simulink model "GTPR_OpenLoop"  (R2021a)
settings: Solver=ode4  StartTime=0.0  StopTime=t_end  FixedStep=t_step  RelTol=1e-3  AbsTol=1e-3
model workspace (MAT data in the model file):
  dt_planner = 0.001
  dt_solver = 0.0002
values from neighbouring files (symbols this model uses):
  aA = 0.5    [SimMechanics_GTPR_OpenLoop_CircularMotion_VS_ClosedLoop.m]
  aB = 0.5    [SimMechanics_GTPR_OpenLoop_CircularMotion_VS_ClosedLoop.m]
  aC = 0.5    [SimMechanics_GTPR_OpenLoop_CircularMotion_VS_ClosedLoop.m]
  dq_init = dq_des_c(:,1)    [SimMechanics_GTPR_OpenLoop_CircularMotion_VS_ClosedLoop.m]
  eA = 0.28    [SimMechanics_GTPR_OpenLoop_CircularMotion_VS_ClosedLoop.m]
  eB = 0.28    [SimMechanics_GTPR_OpenLoop_CircularMotion_VS_ClosedLoop.m]
  eC = 0.28    [SimMechanics_GTPR_OpenLoop_CircularMotion_VS_ClosedLoop.m]
  ILA = zeros(3)    [SimMechanics_GTPR_OpenLoop_CircularMotion_VS_ClosedLoop.m]
  IlA = zeros(3)    [SimMechanics_GTPR_OpenLoop_CircularMotion_VS_ClosedLoop.m]
  ILB = zeros(3)    [SimMechanics_GTPR_OpenLoop_CircularMotion_VS_ClosedLoop.m]
  IlB = zeros(3)    [SimMechanics_GTPR_OpenLoop_CircularMotion_VS_ClosedLoop.m]
  ILC = zeros(3)    [SimMechanics_GTPR_OpenLoop_CircularMotion_VS_ClosedLoop.m]
  q_init = q_des_c(:,1)    [SimMechanics_GTPR_OpenLoop_CircularMotion_VS_ClosedLoop.m]
  t_step = 0.001    [SimMechanics_GTPR_OpenLoop_CircularMotion_VS_ClosedLoop.m]
libraries: nesl_utility x22, sm_lib x3, GTPR_Library x1
CloseFcn:
  | clear sm_pick_and_place_robot_ik
  | clear sm_pick_and_place_robot_fk
Description:
  | Pick and Place Robot with Forward and Inverse Kinematics
settings Model: Creator=The MathWorks, Inc.  LastModifiedBy=szucs
settings SolverCC: NumberNewtonIterations=100  AlgebraicLoopSolver=TrustRegion
settings DataIOCC: ReturnWorkspaceOutputs=off
settings DebuggingCC: SFMachineParentedDataDiag=warning
settings SimscapeCC: SimscapeLogType=all  SimscapeLogSimulationStatistics=on  SimscapeLogName=simlog_sm_pick_and_place_robot  SimscapeLogDataHistory=10000
settings ExplorerConfigSet: InternalSimMechanicsExplorerSettings="<ExplorerConfiguration><canonicalview>default</canonicalview><AnimationSetting><BasePlaybackSpeed>1.0</BasePlaybackSpeed><PlaybackSpeedFactor>1.0</PlaybackSpeedFactor></AnimationSetting><TilePanel><TileInfo><Tiles Columns=\"2\" Count=\"3\" Rows=\"2\"><Column Weight=\"0.5\"/><Column Weight=\"0.5\"/><Row Weight=\"0.3038\"/><Row Weight=\"0.6962\"/><Tile Height=\"2\" Width=\"1\" X=\"0\" Y=\"0\"/><Tile Height=\"1\" Width=\"1\" X=\"1\" Y=\"0\"/><Tile Height=\"1\" Width=\"1\" X=\"1\" Y=\"1\"/></Tiles></TileInfo><SceneInfo><SceneViewer><BGColor><R>0.60000002384185791</R><G>0.60000002384185791</G><B>0.60000002384185791</B></BGColor><Camera><DoPerspective>off</DoPerspective><Position><X>0.674555883500480347</X><Y>-0.674555883500480902</Y><Z>0.921885249943208973</Z></Position><Center><X>0.0060149771328419227</X><Y>-0.00601497713284246394</Y><Z>0.253344343575570674</Z></Center><Up><X>-0.408248290463863073</X><Y>0.408248290463863073</Y><Z>0.816496580927726145</Z></Up><ViewLimDist>1</ViewLimDist><YLim>0.43506960332393646</YLim><XLim>0.392966093324845833</XLim></Camera></SceneViewer><SceneViewer><BGColor><R>0.60000002384185791</R><G>0.60000002384185791</G><B>0.60000002384185791</B></BGColor><Camera><DoPerspective>off</DoPerspective><Position><X>-0.000385309004919674389</X><Y>-1.33915517216324798</Y><Z>0.0518624305243804845</Z></Position><Center><X>-0.000385309004919674389</X><Y>0.0454699993133544367</Y><Z>0.0518624305243804845</Z></Center><Up><X>0</X><Y>-0</Y><Z>1</Z></Up><ViewLimDist>1</ViewLimDist><YLim>0.0894075615531887413</YLim><XLim>0.282074560393158813</XLim></Camera></SceneViewer><SceneViewer><BGColor><R>0.60000002384185791</R><G>0.60000002384185791</G><B>0.60000002384185791</B></BGColor><Camera><DoPerspective>on</DoPerspective><Position><X>-1.13755508710961844e-18</X><Y>-8.63362207815730793e-18</Y><Z>0.589999999999999969</Z></Position><Center><X>-1.13755508710961844e-18</X><Y>-8.63362207815730793e-18</Y><Z>-0.410000000000000031</Z></Center><Up><X>0</X><Y>1</Y><Z>0</Z></Up><ViewLimDist>1</ViewLimDist><YLim>0.466307658154998583</YLim><XLim>0.621743544206664778</XLim></Camera></SceneViewer></SceneInfo></TilePanel><MechEditorPanel><Cameras><Camera><Id>Camera1</Id><Value><Name>CameraView</Name><NativeCamera><PositionTrackingFeature>Delta_Robot.Camera_Frame</PositionTrackingFeature><CenterTrackingFeature>Delta_Robot.Camera_Frame</CenterTrackingFeature><UpVectorTrackingFeature>Delta_Robot.Camera_Frame</UpVectorTrackingFeature><CenterTrackingOrigin>off</CenterTrackingOrigin><CenterTrackingDirection>+Z</CenterTrackingDirection><UpVectorTrackingDirection>-Y</UpVectorTrackingDirection></NativeCamera></Value></Camera></Cameras><GfxPanelCameraMap><MapElement CameraMLId=\"Camera1\" GfxPanelIndex=\"2\"/></GfxPanelCameraMap><VideoCreator><PlaybackSpeedRatio>1.0</PlaybackSpeedRatio><FrameRate>30</FrameRate><VideoFormat>Motion JPEG AVI</VideoFormat><FrameSize>auto</FrameSize></VideoCreator></MechEditorPanel></ExplorerConfiguration>"

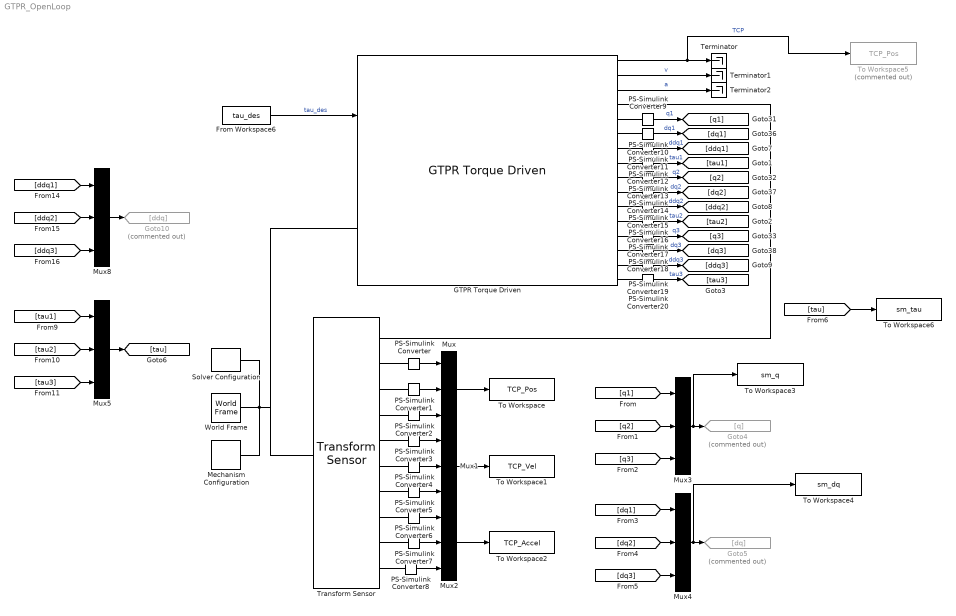
== system GTPR_OpenLoop ==
  From Workspace6 : FromWorkspace  VariableName=tau_des  OutDataTypeStr=double  SampleTime=t_step  OutputAfterFinalValue=Holding final value
  GTPR Torque Driven : GTPR_Library/GTPR Torque Driven  q1=q_init(1)  q2=q_init(2)  q3=q_init(3)  dq1=dq_init(1)  dq2=dq_init(2)  dq3=dq_init(3)  LengthUpperA=LA  LengthLowerA=lA  LengthLinkA=0.1  RadiusUpperA=0.01  RadiusLowerA=0.01  RadiusLinkA=0.01  RadiusCoverA=0.02  MassUpperA=mLA  MassLowerA=mlA  MassLinkA=m_unaccounted  ColorA=[1, 0, 0]  IA_Upper_xx=ILA(1,1)  IA_Upper_xy=ILA(1,2)  IA_Upper_xz=ILA(1,3)  IA_Upper_yy=ILA(2,2)  IA_Upper_yz=ILA(2,3)  IA_Upper_zz=ILA(3,3)  IA_Lower_xx=IlA(1,1)  IA_Lower_xy=IlA(1,2)  IA_Lower_xz=IlA(1,3)  IA_Lower_yy=IlA(2,2)  IA_Lower_yz=IlA(2,3)  IA_Lower_zz=IlA(3,3)  LengthUpperB=LB  LengthLowerB=lB  LengthLinkB=0.1  RadiusUpperB=0.01  RadiusLowerB=0.01  RadiusLinkB=0.01  RadiusCoverB=0.02  MassUpperB=mLB  MassLowerB=mlB  MassLinkB=m_unaccounted  ColorB=[0, 1, 0]  IB_Upper_xx=ILB(1,1)  IB_Upper_xy=ILB(1,2)  IB_Upper_xz=ILB(1,3)  IB_Upper_yy=ILB(2,2)  IB_Upper_yz=ILB(2,3)  IB_Upper_zz=ILB(3,3)  IB_Lower_xx=IlB(1,1)  IB_Lower_xy=IlB(1,2)  IB_Lower_xz=IlB(1,3)  IB_Lower_yy=IlB(2,2)  IB_Lower_yz=IlB(2,3)  IB_Lower_zz=IlB(3,3)  LengthUpperC=LC  LengthLowerC=lC  LengthLinkC=0.1  RadiusUpperC=0.01  RadiusLowerC=0.01  RadiusLinkC=0.01  RadiusCoverC=0.02  MassUpperC=mLC  MassLowerC=mlC  MassLinkC=m_unaccounted  ColorC=[0, 0, 1]  IC_Upper_xx=ILC(1,1)  IC_Upper_xy=ILC(1,2)  IC_Upper_xz=ILC(1,3)  IC_Upper_yy=ILC(2,2)  IC_Upper_yz=ILC(2,3)  IC_Upper_zz=ILC(3,3)  IC_Lower_xx=ILC(1,1)  IC_Lower_xy=ILC(1,2)  IC_Lower_xz=ILC(1,3)  IC_Lower_yy=ILC(2,2)  IC_Lower_yz=ILC(2,3)  IC_Lower_zz=ILC(3,3)  DistBaseA=aA  DistBaseB=aB  DistBaseC=aC  Rtop=max([aA, aB, aC])  DistWorkA=eA  DistWorkB=eB  DistWorkC=eC  MassTCP=mTCP  Rbot=max([eA, eB, eC])  NoOfSides=6  alphaAB=alphaAB  alphaAC=alphaAC
      settings: SourceProductName=Generalized Triangle Parallel Robot
  Goto10 : Goto  Commented=on  GotoTag=ddq
  Goto4 : Goto  Commented=on  GotoTag=q
  Goto5 : Goto  Commented=on  GotoTag=dq
  Mechanism Configuration : sm_lib/Utilities/Mechanism Configuration  UniformGravity=Constant  GravityVector=[0 0 -9.80665]  GravityVectorUnits=m/s^2  GravityUnits=m/s^2  LinearizationDelta=t_step/10  JointModeTransitionNonlinearIterations=30
  Mux{,1..5,8} (7 alike) : Mux  Inputs=3
  PS-Simulink Converter{,1..20} (21 alike) : nesl_utility/PS-Simulink Converter  PhysicalDomain=network_engine_domain  SubClassName=ps_output  LeftPortType=input  RightPortType=output  PseudoPeriodic=off  Frequencies=[]  Unit=inherit  AffineConversion=off
      settings: SourceProductBaseCode=PW,SS
  Solver Configuration : nesl_utility/Solver Configuration  PhysicalDomain=network_engine_domain  SubClassName=solver  LeftPortType=input  RightPortType=generic  Tones=[]  Harmonics=[]  SimulateNoise=off  Profile=off  UseLocalSampling=off  EnableSwitchedLinearOptims=on  FrequencyDomain=off  UseCCode=off  RelTol=0.001  AbsTol=1e-06  MinStep=1e-09  ToWorkspace=off  RevertToSquareIcSolve=off  NumHomotopyIterations=100  PhasorMode=off  PhasorModeNumHarmonics=1  DoDC=off  ResidualTolerance=1e-10  UseLocalSolver=off  LocalSolverChoice=NE_BACKWARD_EULER_ADVANCER  LocalSolverSampleTime=0.001  DoFixedCost=off  MaxNonlinIter=3  MaxModeIter=2  ComputeImpulses=off  ImpulseIterations=2  LinearAlgebra=Full  EquationFormulation=NE_FREQUENCY_TIME_EF  DelaysMemoryBudget=1024  AutomaticFiltering=on  FilteringTimeConstant=t_step/10  PartitionStorageMethod=AS_NEEDED  PartitionMemoryBudget=1024  PartitionMethod=FAST
      settings: SourceProductBaseCode=PW,SS
  Terminator : Terminator
  Terminator1 : Terminator
  Terminator2 : Terminator
  To Workspace : ToWorkspace  VariableName=TCP_Pos  SaveFormat=Timeseries  SampleTime=t_step
  To Workspace1 : ToWorkspace  VariableName=TCP_Vel  SaveFormat=Timeseries  SampleTime=t_step
  To Workspace2 : ToWorkspace  VariableName=TCP_Accel  SaveFormat=Timeseries  SampleTime=t_step
  To Workspace3 : ToWorkspace  VariableName=sm_q  SaveFormat=Timeseries  SampleTime=t_step
  To Workspace4 : ToWorkspace  VariableName=sm_dq  SaveFormat=Timeseries  SampleTime=t_step
  To Workspace5 : ToWorkspace  Commented=on  VariableName=TCP_Pos  SaveFormat=Timeseries  SampleTime=-1
  To Workspace6 : ToWorkspace  VariableName=sm_tau  SaveFormat=Timeseries  SampleTime=t_step
  Transform Sensor : sm_lib/Frames and Transforms/Transform Sensor  MeasurementFrame=World  SenseAngle=off  SenseAxis=off  SenseAngle1=off  SenseAngle2=off  SenseAngle3=off  SenseQ=off  SenseR=off  SenseOmegaX=off  SenseOmegaY=off  SenseOmegaZ=off  SenseOmega1=off  SenseOmega2=off  SenseOmega3=off  SenseQDot=off  SenseRDot=off  SenseAlphaX=off  SenseAlphaY=off  SenseAlphaZ=off  SenseAlpha1=off  SenseAlpha2=off  SenseAlpha3=off  SenseQDDot=off  SenseRDDot=off  SenseX=on  SenseY=on  SenseZ=on  SenseRad=off  SenseAzim=off  SenseDist=off  SenseInc=off  SenseXDot=on  SenseYDot=on  SenseZDot=on  SenseRadDot=off  SenseAzimDot=off  SenseDistDot=off  SenseIncDot=off  SenseXDDot=on  SenseYDDot=on  SenseZDDot=on  SenseRadDDot=off  SenseAzimDDot=off  SenseDistDDot=off  SenseIncDDot=off
  World Frame : sm_lib/Frames and Transforms/World Frame
  wires:
  PS-Simulink Converter1/1 -> Mux/2
  PS-Simulink Converter/1 -> Mux/1
  PS-Simulink Converter2/1 -> Mux/3
  PS-Simulink Converter3/1 -> Mux1/1
  PS-Simulink Converter4/1 -> Mux1/2
  PS-Simulink Converter5/1 -> Mux1/3
  PS-Simulink Converter6/1 -> Mux2/1
  PS-Simulink Converter7/1 -> Mux2/2
  PS-Simulink Converter8/1 -> Mux2/3
  Mux/1 -> To Workspace/1
  Mux1/1 -> To Workspace1/1
  Mux2/1 -> To Workspace2/1
  PS-Simulink Converter13/1 -> [q2]  "q2"
  PS-Simulink Converter9/1 -> [q1]  "q1"
  PS-Simulink Converter17/1 -> [q3]  "q3"
  PS-Simulink Converter10/1 -> [dq1]  "dq1"
  PS-Simulink Converter14/1 -> [dq2]  "dq2"
  PS-Simulink Converter18/1 -> [dq3]  "dq3"
  [q1] -> Mux3/1
  [q2] -> Mux3/2
  [q3] -> Mux3/3
  Mux3/1 -> To Workspace3/1, Goto4/1
  [dq2] -> Mux4/2
  [dq1] -> Mux4/1
  [dq3] -> Mux4/3
  Mux4/1 -> To Workspace4/1, Goto5/1
  GTPR Torque Driven/1 -> To Workspace5/1, Terminator/1  "TCP"
  GTPR Torque Driven/2 -> Terminator1/1  "v"
  GTPR Torque Driven/3 -> Terminator2/1  "a"
  PS-Simulink Converter12/1 -> [tau1]  "tau1"
  PS-Simulink Converter16/1 -> [tau2]  "tau2"
  PS-Simulink Converter20/1 -> [tau3]  "tau3"
  [tau2] -> Mux5/2
  [tau1] -> Mux5/1
  Mux5/1 -> [tau]
  [tau3] -> Mux5/3
  PS-Simulink Converter11/1 -> [ddq1]  "ddq1"
  PS-Simulink Converter15/1 -> [ddq2]  "ddq2"
  PS-Simulink Converter19/1 -> [ddq3]  "ddq3"
  [ddq2] -> Mux8/2
  [ddq1] -> Mux8/1
  Mux8/1 -> Goto10/1
  [ddq3] -> Mux8/3
  [tau] -> To Workspace6/1
  From Workspace6/1 -> GTPR Torque Driven/1  "tau_des"
  connections:
  World Frame/RConn1 -- GTPR Torque Driven/LConn1 -- Transform Sensor/LConn1 -- Solver Configuration/RConn1 -- Mechanism Configuration/RConn1
  Transform Sensor/RConn1 -- GTPR Torque Driven/RConn1
  PS-Simulink Converter/LConn1 -- Transform Sensor/RConn2
  PS-Simulink Converter1/LConn1 -- Transform Sensor/RConn3
  PS-Simulink Converter2/LConn1 -- Transform Sensor/RConn4
  PS-Simulink Converter3/LConn1 -- Transform Sensor/RConn5
  PS-Simulink Converter4/LConn1 -- Transform Sensor/RConn6
  Transform Sensor/RConn7 -- PS-Simulink Converter5/LConn1
  Transform Sensor/RConn8 -- PS-Simulink Converter6/LConn1
  Transform Sensor/RConn9 -- PS-Simulink Converter7/LConn1
  Transform Sensor/RConn10 -- PS-Simulink Converter8/LConn1
  PS-Simulink Converter9/LConn1 -- GTPR Torque Driven/RConn2
  PS-Simulink Converter10/LConn1 -- GTPR Torque Driven/RConn3
  PS-Simulink Converter11/LConn1 -- GTPR Torque Driven/RConn4
  PS-Simulink Converter12/LConn1 -- GTPR Torque Driven/RConn5
  GTPR Torque Driven/RConn7 -- PS-Simulink Converter14/LConn1
  GTPR Torque Driven/RConn6 -- PS-Simulink Converter13/LConn1
  GTPR Torque Driven/RConn8 -- PS-Simulink Converter15/LConn1
  GTPR Torque Driven/RConn10 -- PS-Simulink Converter17/LConn1
  GTPR Torque Driven/RConn9 -- PS-Simulink Converter16/LConn1
  GTPR Torque Driven/RConn11 -- PS-Simulink Converter18/LConn1
  GTPR Torque Driven/RConn13 -- PS-Simulink Converter20/LConn1
  GTPR Torque Driven/RConn12 -- PS-Simulink Converter19/LConn1
